simulink model "arduino_pil_block_2016a"  (R2016a)
settings: Solver=ode3  StartTime=0.0  StopTime=10  FixedStep=0.01  RelTol=1e-3
Description:
  | Software-in-the-Loop Code Verification
settings Model: ModifiedByFormat=The MathWorks Inc.  SimulationMode=processor-in-the-loop (pil)  ExtModeTrigDuration=2  ExtModeAutoUpdateStatusClock=off  Creator=The MathWorks, Inc.  LastModifiedBy=The MathWorks Inc.
settings SolverCC: PositivePriorityOrder=on
settings DataIOCC: SaveFormat=Array  SignalLogging=off  ReturnWorkspaceOutputs=on  SignalLoggingName=sigsOut
settings OptimizationCC: UseDivisionForNetSlopeComputation=UseDivisionForReciprocalsOfIntegersOnly  EnhancedBackFolding=on  BooleansAsBitfields=on  PassReuseOutputArgsAs=Individual arguments  ExpressionDepthLimit=2147483647  StateBitsets=on  DataBitsets=on  ZeroExternalMemoryAtStartup=off  ZeroInternalMemoryAtStartup=off  NoFixptDivByZeroProtection=on  EfficientFloat2IntCast=on  OptimizeModelRefInitCode=on  LifeSpan=1  MaxStackSize=64
settings DebuggingCC: CheckExecutionContextPreStartOutputMsg=on  CheckExecutionContextRuntimeOutputMsg=on  FcnCallInpInsideContextMsg=EnableAllAsWarning  UnconnectedLineMsg=none  AllowSymbolicDim=off  StateNameClashWarn=warning  StrictBusMsg=ErrorOnBusTreatedAsVector
settings HardwareCC: ProdBitPerInt=16  ProdBitPerPointer=16  ProdLargestAtomicFloat=None  ProdWordSize=8  ProdHWDeviceType=Atmel->AVR  TargetBitPerPointer=64  TargetLongLongMode=on  TargetIntDivRoundTo=Zero  TargetEndianess=LittleEndian  TargetWordSize=64  TargetHWDeviceType=Generic->MATLAB Host Computer
settings ModelReferenceCC: PropagateSignalLabelsOutOfModel=off
settings RTWCC: SystemTargetFile=ert.tlc  HardwareBoard=Arduino Uno  TemplateMakefile=ert_default_tmf  GenerateReport=on  RTWVerbose=off  Toolchain=Arduino AVR  BuildConfiguration=Faster Runs  IncludeHyperlinkInReport=on  PortableWordSizes=on  CreateSILPILBlock=PIL  GenerateTraceInfo=on  GenerateTraceReport=on  GenerateTraceReportSl=on  GenerateTraceReportSf=on  GenerateTraceReportEml=on  GenerateCodeMetricsReport=on
settings CodeAppCC: ForceParamTrailComments=on  IgnoreCustomStorageClasses=off  IgnoreTestpoints=on  SimulinkDataObjDesc=on  CustomSymbolStrGlobalVar=rt$N$M  CustomSymbolStrType=$N$M  CustomSymbolStrFcn=$N$M$F  CustomSymbolStrMacro=$N$M  InsertBlockDesc=on  InternalIdentifier=Classic
settings ERTTargetCC: UtilityFuncGeneration=Shared location  IncludeMdlTerminateFcn=off  CombineSignalStateStructs=on  SupportNonFinite=off  SupportComplex=off  SupportContinuousTime=on  SupportVariableSizeSignals=on  ERTFilePackagingFormat=CompactWithDataFile  ConvertIfToSwitch=off  SuppressUnreachableDefaultCases=off
settings ConfigComp: CovSFcnEnable=off

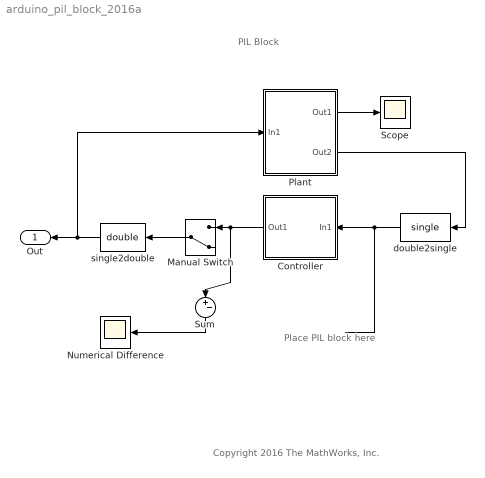
== system arduino_pil_block_2016a ==
  note: Place PIL
      | block here
  note: Copyright 2016 The MathWorks, Inc.
  note: PIL Block
  Controller : Subsystem  TreatAsAtomicUnit=on
      settings: RTWFcnNameOpts=Use subsystem name  RTWFileNameOpts=Use function name
  Manual Switch : ManualSwitch  CurrentSetting=0
  Numerical Difference : Scope
  Plant : Subsystem
  Scope : Scope
  Sum : Sum  Inputs=|+-
  double2single : DataTypeConversion  OutDataTypeStr=single
  single2double : DataTypeConversion  OutDataTypeStr=double
  Out : Outport
  wires:
  Plant/1(Out1) -> Scope/1
  Plant/2(Out2) -> double2single/1
  double2single/1 -> Controller/1(In1)
  single2double/1 -> Plant/1(In1), Out/1
  Controller/1(Out1) -> Sum/1, Manual Switch/1
  Manual Switch/1 -> single2double/1
  ? -> Sum/2, Manual Switch/2
  Sum/1 -> Numerical Difference/1

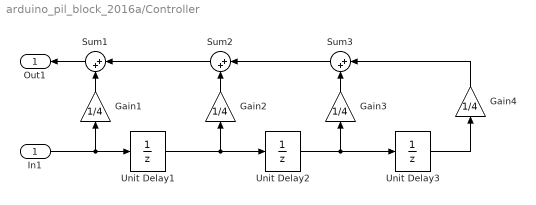
== system arduino_pil_block_2016a/Controller ==
  In1 : Inport  SampleTime=.01
  Gain{1..4} (4 alike) : Gain  Gain=1/4  SaturateOnIntegerOverflow=on  ParamDataTypeStr=Inherit: Same as input
  Sum1 : Sum  Inputs=|++  SaturateOnIntegerOverflow=on  InputSameDT=on  OutDataTypeStr=Inherit: Same as first input
  Sum2 : Sum  Inputs=|++  SaturateOnIntegerOverflow=on  InputSameDT=on  OutDataTypeStr=Inherit: Same as first input
  Sum3 : Sum  Inputs=|++  SaturateOnIntegerOverflow=on  InputSameDT=on  OutDataTypeStr=Inherit: Same as first input
  Unit Delay1 : UnitDelay  SampleTime=-1
  Unit Delay2 : UnitDelay  SampleTime=-1
  Unit Delay3 : UnitDelay  SampleTime=-1
  Out1 : Outport
  wires:
  Gain1/1 -> Sum1/2
  In1/1 -> Unit Delay1/1, Gain1/1
  Sum1/1 -> Out1/1
  Sum3/1 -> Sum2/1
  Sum2/1 -> Sum1/1
  Unit Delay1/1 -> Unit Delay2/1, Gain2/1
  Unit Delay2/1 -> Unit Delay3/1, Gain3/1
  Unit Delay3/1 -> Gain4/1
  Gain4/1 -> Sum3/1
  Gain3/1 -> Sum3/2
  Gain2/1 -> Sum2/2

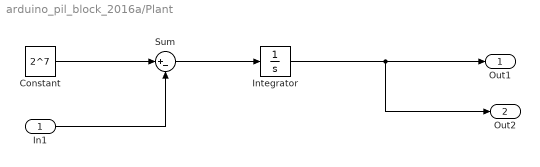
== system arduino_pil_block_2016a/Plant ==
  In1 : Inport
  Constant : Constant  Value=2^7
  Integrator : Integrator
  Sum : Sum  Inputs=|+-  SaturateOnIntegerOverflow=on  InputSameDT=on  OutDataTypeStr=Inherit: Same as first input
  Out1 : Outport
  Out2 : Outport  Port=2
  wires:
  Integrator/1 -> Out1/1, Out2/1
  Sum/1 -> Integrator/1
  Constant/1 -> Sum/1
  In1/1 -> Sum/2
